simulink model "test"  (R2021a)
settings: Solver=FixedStepDiscrete  StartTime=0.0  StopTime=10.0  FixedStep=0.01  RelTol=1e-3
undefined symbols (not defined in the file): DiscIntNeverNeededParam
libraries: simulink x1
settings Model: Creator=iris  LastModifiedBy=iris

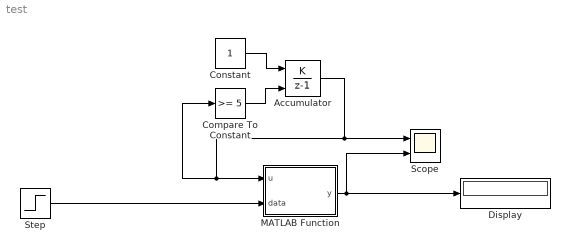
== system test ==
  Accumulator : DiscreteIntegrator  IntegratorMethod=Accumulation: Forward Euler  ExternalReset=rising  SampleTime=-1  ICPrevOutput=DiscIntNeverNeededParam  ICPrevScaledInput=DiscIntNeverNeededParam
  Compare To Constant : simulink/Logic and Bit Operations/Compare To Constant  relop=>=  const=5  OutDataTypeStr=boolean
  Constant : Constant
  Display : Display
  MATLAB Function : MATLAB Function  TreatAsAtomicUnit=on
  Scope : Scope  NumInputPorts=2
  Step : Step  Before=[0 0 0]  After=[1 1 1]  SampleTime=0
  wires:
  Constant/1 -> Accumulator/1
  Accumulator/1 -> Scope/1, MATLAB Function/1(u), Compare To Constant/1
  Compare To Constant/1 -> Accumulator/2
  Step/1 -> MATLAB Function/2(data)
  MATLAB Function/1(y) -> Scope/2, Display/1

== matlab function test/MATLAB Function ==
  data: u input; y output; data input
function y= fcn(u, data)


persistent please_do_it


if isempty(please_do_it)
    please_do_it = zeros(5,3);
end

please_do_it(u+1,:)=data;
y = please_do_it;

end
